simulink model "MKF_example_sim"  (R2021b)
settings: Solver=FixedStepAuto  StartTime=0.0  StopTime=nT*Ts  FixedStep=Ts  RelTol=1e-3
values from neighbouring files (symbols this model uses):
  A = Model.A    [GPB1_estimation.m]    (also in GPB2_estimation.m; MKFObserverRODD.m = repmat({A}, 1, nj); MKFObserverSF.m = repmat({A}, 1, nj); MKFObserverSF95.m = repmat({A}, 1, nj))
  B = Model.B    [GPB1_estimation.m]    (also in GPB2_estimation.m)
  Bu = repmat({Bu}, 1, nj)    [MKFObserverRODD.m]    (also in MKFObserverSF.m; MKFObserverSF95.m; MKFObserverSF98.m; MKFObserverSF_RODD.m = model.B(:, u_meas))
  C = Model.C    [GPB1_estimation.m]    (also in GPB2_estimation.m; MKFObserverDI.m = obj.filters{f}.C; MKFObserverF.m = obj.filters{f}.C; MKFObserverGPB1.m = obj.filters{f}.C)
  Du = repmat({Du}, 1, nj)    [MKFObserverRODD.m]    (also in MKFObserverSF.m; MKFObserverSF95.m; MKFObserverSF_RODD.m = model.D(:, u_meas))
  x0 = zeros(n, 1)    [AbstractLinearFilter.m]    (also in EKF_filter.m; EKF_observer.m; KalmanFilter.m; KalmanFilterJS.m = zeros(obj.n, 1))
undefined symbols (not defined in the file or in its folder): Discrete, KF1, KFSS, MKF1, MKF2, Time, Ts
libraries: ctrlSharedLib x1
settings Model: Creator=Andre  LastModifiedBy=billtubbs
settings SolverCC: AlgebraicLoopSolver=TrustRegion
settings DataIOCC: ReturnWorkspaceOutputs=off
settings DebuggingCC: SFMachineParentedDataDiag=warning  ArithmeticOperatorsInVariantConditions=warning
settings SFSimCC: SimUseLocalCustomCode=off  CustomCodeUndefinedFunction=UseInterfaceOnly
settings RTWCC: RTWUseLocalCustomCode=off

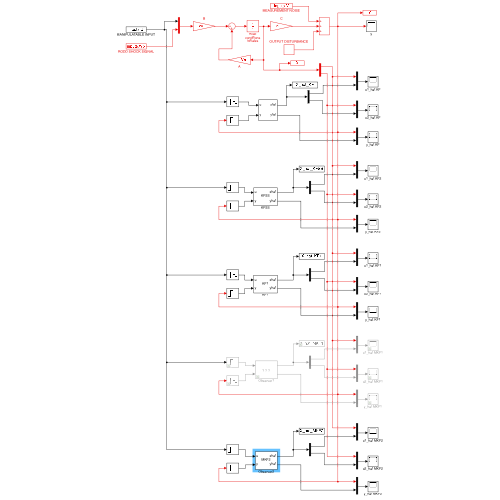
[thumbnail: Simulink's stored preview of the top-level diagram]
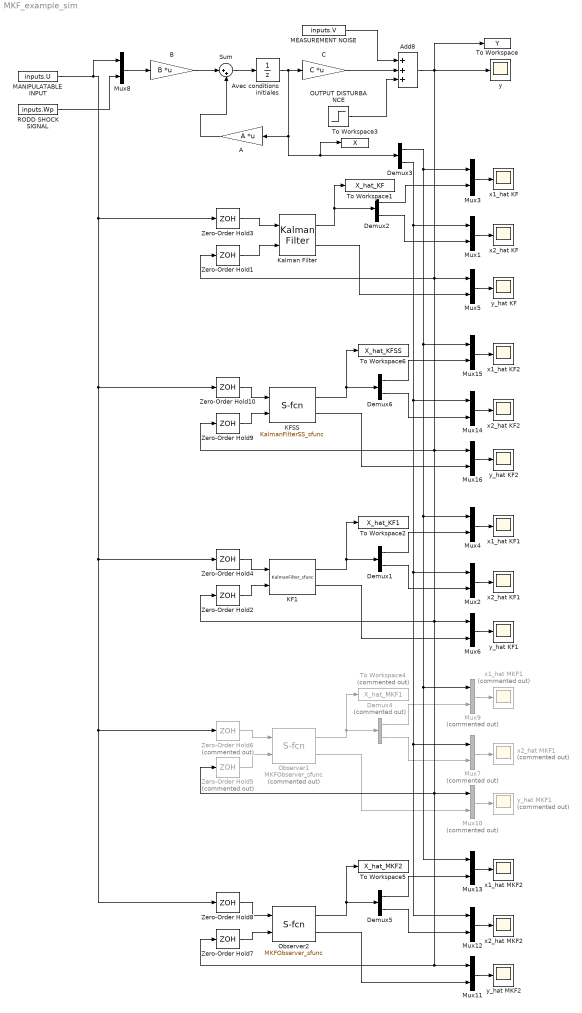
== system MKF_example_sim ==
  A : Gain  Gain=A  Multiplication=Matrix(K*u)
  Add8 : Sum  Inputs=+++
  Avec conditions initiales : UnitDelay  InitialCondition=x0  SampleTime=Ts  HasFrameUpgradeWarning=on
  B : Gain  Gain=B  Multiplication=Matrix(K*u)
  C : Gain  Gain=C  Multiplication=Matrix(K*u)
  Demux{1..3,5..6} (5 alike) : Demux  Outputs=2
  Demux4 : Demux  Commented=on  Outputs=2
  KF1 : M-S-Function  FunctionName=KalmanFilter_sfunc  Parameters=obs  mask{obs=KF1}
      mask prompts: obs "Observer"
      mask help:
      | Kalman Filter
      |
      | Inputs:
      |  - u : measured process inputs
      |  - y : measured process outputs
      |
      | Outputs:
      |  - xhat : estimate of process states in next time step
      |  - yhat : estimate of process outputs in next time step
      mask Help:
      | <h1>Kalman Filter</h1>
      | 
      | Inputs:
      | <ol>
      | <li>u : measured process inputs (<code>uk</code> argument of update_KF function)
      | <li>y : measured process outputs (<code>yk</code> argument of update_KF function)
      | </ol>
      | 
      | Outputs:
      | <ol>
      | <li>xhat : estimate of process states in next time step (<code>xkp1_est</code> attribute of obs struct)
      | <li>yhat : estimate of process outputs in next time step (<code>ykp1_est</code> of obs struct)
      | </ol>
      | 
      | Use this block to simulate process observers generated by the following MATLAB functions:
      | <ul>
      | <li><code>kalman_filter</code>
      | <li><code>kalman_filter_ss</code>
      | <li><code>luenberger_observer</code>
      | </ul>
      | 
      | <h2>Instructions</h2>
      | 
      | First, generate the observer struct in the MATLAB workspace then pass it to this block in the input field in the block mask. The simulink block will then simulate the observer.  Note that the original MATLAB observer struct will not be updated with the states from the simulation.
      | 
      | The s-functions which can be used with this block:
      | <ul>
      | <li><code>kalman_filter_sfunc</code>
      | <li><code>kalman_filter_ss_sfunc</code>
      | </ul>
      | 
      | To change the s-function, select Mask > Look Under Mask and edit the function name.
      | 
      | <h2>Code repository</h2>
      | <ul>
      | <li><a href="https://github.com/billtubbs/process-observers">https://github.com/billtubbs/process-observers</a>
      | </ul>
      mask Display:
      | port_label('input', 1, 'u')
      | port_label('input', 2, 'y')
      | port_label('output', 1, 'xhat')
      | port_label('output', 2, 'yhat')
      | disp(obs.label)
  KFSS : M-S-Function  FunctionName=KalmanFilterSS_sfunc  Parameters=obs  mask{obs=KFSS}
      mask prompts: obs "Observer"
      mask help:
      | Kalman Filter
      |
      | Inputs:
      |  - u : measured process inputs
      |  - y : measured process outputs
      |
      | Outputs:
      |  - xhat : estimate of process states in next time step
      |  - yhat : estimate of process outputs in next time step
      mask Help:
      | <h1>Kalman Filter</h1>
      | 
      | Inputs:
      | <ol>
      | <li>u : measured process inputs (<code>uk</code> argument of update_KF function)
      | <li>y : measured process outputs (<code>yk</code> argument of update_KF function)
      | </ol>
      | 
      | Outputs:
      | <ol>
      | <li>xhat : estimate of process states in next time step (<code>xkp1_est</code> attribute of obs struct)
      | <li>yhat : estimate of process outputs in next time step (<code>ykp1_est</code> of obs struct)
      | </ol>
      | 
      | Use this block to simulate process observers generated by the following MATLAB functions:
      | <ul>
      | <li><code>kalman_filter</code>
      | <li><code>kalman_filter_ss</code>
      | <li><code>luenberger_observer</code>
      | </ul>
      | 
      | <h2>Instructions</h2>
      | 
      | First, generate the observer struct in the MATLAB workspace then pass it to this block in the input field in the block mask. The simulink block will then simulate the observer.  Note that the original MATLAB observer struct will not be updated with the states from the simulation.
      | 
      | The s-functions which can be used with this block:
      | <ul>
      | <li><code>kalman_filter_sfunc</code>
      | <li><code>kalman_filter_ss_sfunc</code>
      | </ul>
      | 
      | To change the s-function, select Mask > Look Under Mask and edit the function name.
      | 
      | <h2>Code repository</h2>
      | <ul>
      | <li><a href="https://github.com/billtubbs/process-observers">https://github.com/billtubbs/process-observers</a>
      | </ul>
      mask Display:
      | port_label('input', 1, 'u')
      | port_label('input', 2, 'y')
      | port_label('output', 1, 'xhat')
      | port_label('output', 2, 'yhat')
      | disp(obs.label)
  Kalman Filter : ctrlSharedLib/Kalman Filter  TimeDomain=Discrete-Time  UseCurrentEstimator=off  ModelSource=Individual A, B, C, D matrices  ModelSourceVariable=G  A=A  B=Bu  C=C  D=Du  NumberOfStates=1  NumberOfInputs=1  NumberOfOutputs=1  InitialEstimateSource=Dialog  X0=[0; 0]  P0=10  UseK=off  UseGH=off  NumberOfProcessNoiseInputs=1  G=Gkf  TimeInvariantG=on  H=Hkf  TimeInvariantH=on  Q=KF1.model.Q  TimeInvariantQ=on  R=KF1.model.R  TimeInvariantR=on  N=zeros(KF1.n,KF1.ny)  TimeInvariantN=on  AddInputPort=on  AddEnablePort=off  OutputEstimatedY=on  OutputP=off  Ts=KF1.model.Ts
  MANIPULATABLE INPUT : FromWorkspace  VariableName=inputs.U  SampleTime=Ts
  MEASUREMENT NOISE : FromWorkspace  VariableName=inputs.V  SampleTime=Ts
  Mux{1..6,8,11..16} (13 alike) : Mux  Inputs=2
  Mux10 : Mux  Commented=on  Inputs=2
  Mux7 : Mux  Commented=on  Inputs=2
  Mux9 : Mux  Commented=on  Inputs=2
  OUTPUT DISTURBANCE : Step  Time=100  After=0  SampleTime=0
  Observer1 : M-S-Function  Commented=on  FunctionName=MKFObserver_sfunc  Parameters=obs  mask{obs=MKF1}
      mask prompts: obs "Observer"
      mask help:
      | Multi-Model Process Observer
      |
      | Inputs:
      |  - u : measured process inputs
      |  - y : measured process outputs
      |
      | Outputs:
      |  - xhat : estimate of process states in next time step
      |  - yhat : estimate of process outputs in next time step
      mask Help:
      | <h1>Multi-Model Process Observer</h1>
      | 
      | Inputs:
      | <ol>
      | <li>u : measured process inputs (<code>uk</code> argument of update_KF function)
      | <li>y : measured process outputs (<code>yk</code> argument of update_KF function)
      | </ol>
      | 
      | Outputs:
      | <ol>
      | <li>xhat : estimate of process states in next time step (<code>xkp1_est</code> attribute of obs struct)
      | <li>yhat : estimate of process outputs in next time step (<code>ykp1_est</code> of obs struct)
      | </ol>
      | 
      | Use this block to simulate process observers generated by the following MATLAB functions:
      | <ul>
      | <li><code>kalman_filter</code>
      | <li><code>kalman_filter_ss</code>
      | <li><code>luenberger_observer</code>
      | <li><code>mkf_observer</code>
      | <li><code>mkf_observer_RODD</code>
      | <li><code>mkf_observer_AFMM</code>
      | </ul>
      | 
      | <h2>Instructions</h2>
      | 
      | First, generate the observer struct in the MATLAB workspace then pass it to this block in the input field in the block mask. The simulink block will then simulate the observer.  Note that the original MATLAB observer struct will not be updated with the states from the simulation.
      | 
      | The s-function associated with this block is
      | <ul>
      | <li><code>mkf_observer_sfunc</code>
      | </ul>
      | 
      | <h2>Code repository</h2>
      | <ul>
      | <li><a href="https://github.com/billtubbs/process-observers">https://github.com/billtubbs/process-observers</a>
      | </ul>
      mask Display:
      | port_label('input', 1, 'u')
      | port_label('input', 2, 'y')
      | port_label('output', 1, 'xhat')
      | port_label('output', 2, 'yhat')
      | disp(obs.label)
  Observer2 : M-S-Function  FunctionName=MKFObserver_sfunc  Parameters=obs  mask{obs=MKF2}
      mask prompts: obs "Observer"
      mask help:
      | Process Observer
      |
      | Use this block to simulate process observers generated by the following MATLAB functions:
      |  - kalman_filter
      |  - kalman_filter_ss
      |  - luenberger_observer
      |  - mkf_observer
      |  - mkf_observer_RODD
      |  - mkf_observer_AFMM
      mask Help:
      | Process Observer
      | 
      | Use this block to simulate process observers generated by the following MATLAB functions:
      |  - kalman_filter
      |  - kalman_filter_ss
      |  - luenberger_observer
      |  - mkf_observer
      |  - mkf_observer_RODD
      |  - mkf_observer_AFMM
      | 
      | First, generate the observer struct in the MATLAB workspace then pass it to this block in the input field in the block mask. The simulink block will then simulate the observer.  Note that the original MATLAB observer struct will not be updated with the states from the simulation.
      | 
      | The s-function associated with this block is
      |  - mkf_observer_sfunc
      | 
      | Code repository:
      |  - https://github.com/billtubbs/process-observers
      mask Display:
      | port_label('input', 1, 'u')
      | port_label('input', 2, 'y')
      | port_label('output', 1, 'xhat')
      | port_label('output', 2, 'yhat')
      | disp(obs.label)
  RODD SHOCK SIGNAL : FromWorkspace  VariableName=inputs.Wp  SampleTime=Ts
  Sum : Sum  Inputs=|++
  To Workspace : ToWorkspace  VariableName=Y  SaveFormat=Timeseries  SampleTime=-1
  To Workspace1 : ToWorkspace  VariableName=X_hat_KF  SaveFormat=Timeseries  SampleTime=-1
  To Workspace2 : ToWorkspace  VariableName=X_hat_KF1  SaveFormat=Timeseries  SampleTime=-1
  To Workspace3 : ToWorkspace  VariableName=X  SaveFormat=Timeseries  SampleTime=-1
  To Workspace4 : ToWorkspace  Commented=on  VariableName=X_hat_MKF1  SaveFormat=Timeseries  SampleTime=-1
  To Workspace5 : ToWorkspace  VariableName=X_hat_MKF2  SaveFormat=Timeseries  SampleTime=-1
  To Workspace6 : ToWorkspace  VariableName=X_hat_KFSS  SaveFormat=Timeseries  SampleTime=-1
  Zero-Order Hold{1..4,7..10} (8 alike) : ZeroOrderHold  SampleTime=Ts
  Zero-Order Hold5 : ZeroOrderHold  Commented=on  SampleTime=Ts
  Zero-Order Hold6 : ZeroOrderHold  Commented=on  SampleTime=Ts
  x1_hat KF : Scope
  x1_hat KF1 : Scope
  x1_hat KF2 : Scope
  x1_hat MKF1 : Scope  Commented=on
  x1_hat MKF2 : Scope
  x2_hat KF : Scope
  x2_hat KF1 : Scope
  x2_hat KF2 : Scope
  x2_hat MKF1 : Scope  Commented=on
  x2_hat MKF2 : Scope
  y : Scope
  y_hat KF : Scope
  y_hat KF1 : Scope
  y_hat KF2 : Scope
  y_hat MKF1 : Scope  Commented=on
  y_hat MKF2 : Scope
  wires:
  A/1 -> Sum/2
  Mux3/1 -> x1_hat KF/1
  Mux1/1 -> x2_hat KF/1
  Sum/1 -> Avec conditions initiales/1
  B/1 -> Sum/1
  OUTPUT DISTURBANCE/1 -> Add8/3
  C/1 -> Add8/2
  MEASUREMENT NOISE/1 -> Add8/1
  Kalman Filter/2 -> Mux5/2
  Mux5/1 -> y_hat KF/1
  Kalman Filter/1 -> To Workspace1/1, Demux2/1
  Demux2/1 -> Mux3/2
  Demux2/2 -> Mux1/2
  Zero-Order Hold3/1 -> Kalman Filter/1
  Zero-Order Hold1/1 -> Kalman Filter/2
  RODD SHOCK SIGNAL/1 -> Mux8/2
  Mux8/1 -> B/1
  Zero-Order Hold4/1 -> KF1/1
  Zero-Order Hold2/1 -> KF1/2
  Mux6/1 -> y_hat KF1/1
  KF1/2 -> Mux6/2
  Mux4/1 -> x1_hat KF1/1
  Mux2/1 -> x2_hat KF1/1
  KF1/1 -> To Workspace2/1, Demux1/1
  Demux1/1 -> Mux4/2
  Demux1/2 -> Mux2/2
  Avec conditions initiales/1 -> C/1, Demux3/1, To Workspace3/1, A/1
  Demux4/2 -> Mux7/2
  Mux9/1 -> x1_hat MKF1/1
  Observer1/2 -> Mux10/2
  Observer1/1 -> To Workspace4/1, Demux4/1
  Mux7/1 -> x2_hat MKF1/1
  Demux4/1 -> Mux9/2
  Mux10/1 -> y_hat MKF1/1
  Zero-Order Hold6/1 -> Observer1/1
  Zero-Order Hold5/1 -> Observer1/2
  Mux11/1 -> y_hat MKF2/1
  Observer2/1 -> To Workspace5/1, Demux5/1
  Observer2/2 -> Mux11/2
  Mux13/1 -> x1_hat MKF2/1
  Mux12/1 -> x2_hat MKF2/1
  Demux5/1 -> Mux13/2
  Zero-Order Hold8/1 -> Observer2/1
  Demux5/2 -> Mux12/2
  Zero-Order Hold7/1 -> Observer2/2
  Mux16/1 -> y_hat KF2/1
  Demux6/1 -> Mux15/2
  Add8/1 -> To Workspace/1, Mux16/1, Zero-Order Hold9/1, Mux11/1, Zero-Order Hold7/1, Zero-Order Hold5/1, Mux10/1, Zero-Order Hold2/1, Mux6/1, Zero-Order Hold1/1, Mux5/1, y/1
  Mux15/1 -> x1_hat KF2/1
  Demux6/2 -> Mux14/2
  Zero-Order Hold10/1 -> KFSS/1
  KFSS/1 -> To Workspace6/1, Demux6/1
  Mux14/1 -> x2_hat KF2/1
  MANIPULATABLE INPUT/1 -> Mux8/1, Zero-Order Hold10/1, Zero-Order Hold8/1, Zero-Order Hold6/1, Zero-Order Hold4/1, Zero-Order Hold3/1
  KFSS/2 -> Mux16/2
  Demux3/2 -> Mux14/1, Mux12/1, Mux7/1, Mux2/1, Mux1/1
  Zero-Order Hold9/1 -> KFSS/2
  Demux3/1 -> Mux15/1, Mux13/1, Mux9/1, Mux4/1, Mux3/1
